simulink model "tp1auto1"  (R2019a)
settings: Solver=VariableStepAuto  StartTime=0.0  StopTime=10.0  RelTol=1e-3
libraries: simulink x1
settings Model: Creator=mbenahme  LastModifiedBy=mbenahme

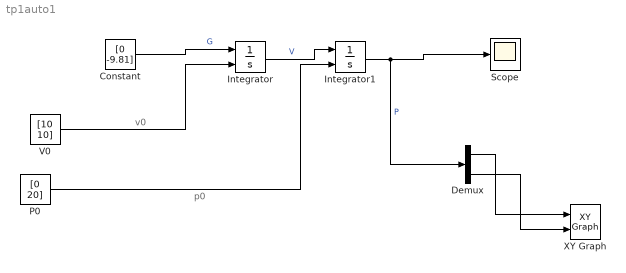
== system tp1auto1 ==
  note: v0
  note: p0
  Constant : Constant  Value=[0 -9.81]
  Demux : Demux  Outputs=2
  Integrator : Integrator  InitialConditionSource=external
  Integrator1 : Integrator  InitialConditionSource=external
  P0 : Constant  Value=[0 20]
  Scope : Scope
  V0 : Constant  Value=[10 10]
  XY Graph : simulink/Sinks/XY Graph  xmin=0  xmax=100  ymin=-400  ymax=50  st=-1
  wires:
  V0/1 -> Integrator/2
  P0/1 -> Integrator1/2
  Integrator/1 -> Integrator1/1  "V"
  Constant/1 -> Integrator/1  "G"
  Integrator1/1 -> Demux/1, Scope/1  "P"
  Demux/2 -> XY Graph/2
  Demux/1 -> XY Graph/1
